simulink model "proiect_model2"  (R2023b)
settings: Solver=VariableStepAuto  StartTime=0.0  StopTime=30  RelTol=1e-3
settings Model: Creator=gabri  LastModifiedBy=gabri

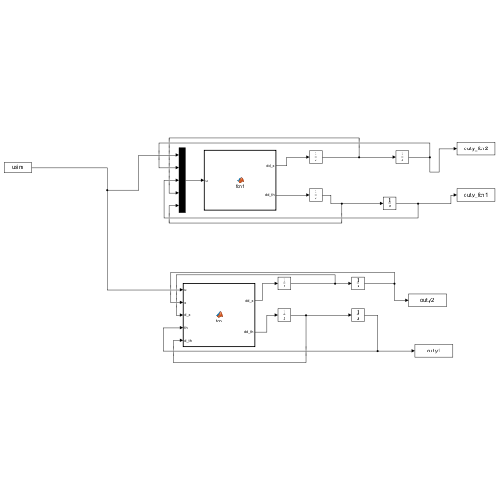
[thumbnail: Simulink's stored preview of the top-level diagram]
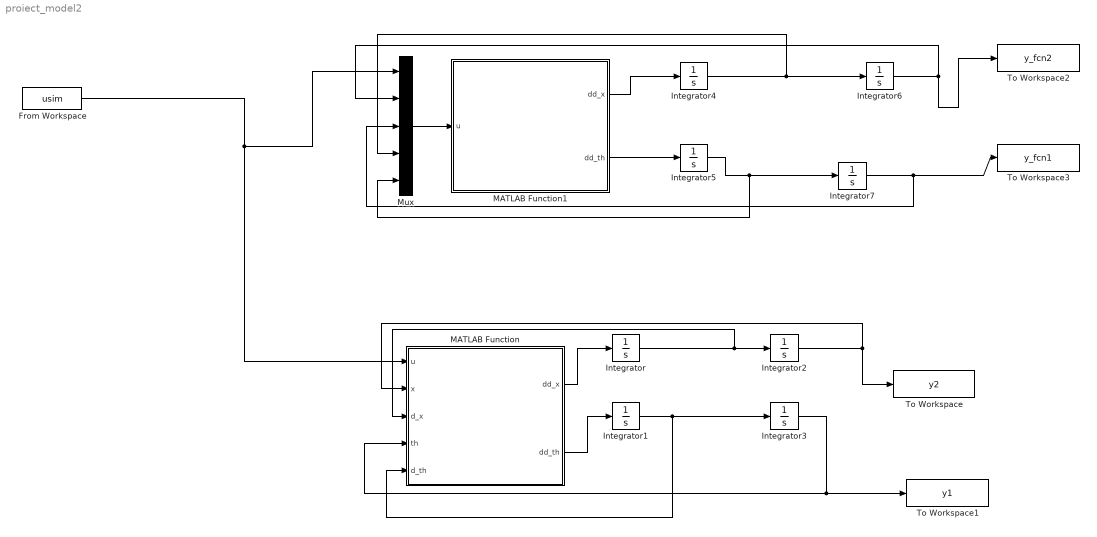
== system proiect_model2 ==
  From Workspace : FromWorkspace  VariableName=usim
  Integrator{,1..7} (8 alike) : Integrator
  MATLAB Function : MATLAB Function  TreatAsAtomicUnit=on
  MATLAB Function1 : MATLAB Function  TreatAsAtomicUnit=on
  Mux : Mux  Inputs=5
  To Workspace : ToWorkspace  VariableName=y2  SaveFormat=Timeseries  SampleTime=-1
      settings: Save2DSignal=2-D array (concatenate along first dimension)
  To Workspace1 : ToWorkspace  VariableName=y1  SaveFormat=Timeseries  SampleTime=-1
      settings: Save2DSignal=2-D array (concatenate along first dimension)
  To Workspace2 : ToWorkspace  VariableName=y_fcn2  SaveFormat=Timeseries  SampleTime=-1
      settings: Save2DSignal=2-D array (concatenate along first dimension)
  To Workspace3 : ToWorkspace  VariableName=y_fcn1  SaveFormat=Timeseries  SampleTime=-1
      settings: Save2DSignal=2-D array (concatenate along first dimension)
  wires:
  Integrator6/1 -> To Workspace2/1, Mux/2
  MATLAB Function/1(dd_x) -> Integrator/1
  Integrator7/1 -> To Workspace3/1, Mux/3
  MATLAB Function1/2(dd_th) -> Integrator5/1
  Mux/1 -> MATLAB Function1/1(u)
  Integrator4/1 -> Integrator6/1, Mux/4
  From Workspace/1 -> Mux/1, MATLAB Function/1(u)
  MATLAB Function1/1(dd_x) -> Integrator4/1
  Integrator5/1 -> Mux/5, Integrator7/1
  Integrator2/1 -> MATLAB Function/2(x), To Workspace/1
  Integrator1/1 -> Integrator3/1, MATLAB Function/5(d_th)
  Integrator3/1 -> To Workspace1/1, MATLAB Function/4(th)
  Integrator/1 -> MATLAB Function/3(d_x), Integrator2/1
  MATLAB Function/2(dd_th) -> Integrator1/1

== matlab function proiect_model2/MATLAB Function1 ==
  data: u input; dd_x output; dd_th output
function [dd_x, dd_th] = fcn1(u)

    %Alegerea valorilor pentru parametrii modelului in mod arbitrar(si pozitiv)
    l0 = 2.42;      %lungimea initiala
    m = 3.53;       %masa corpului   
    k = 3.21;       %constanta elastica
    fact = 0.61;    %factorul de amortizare
    g = 9.81;       %acceleratia gravitationala

    %Formulele modelului
    dd_x = (l0 + u(2)) * (u(5)) * (u(5)) - ((k *u(2)) / m) + g * cos(u(3)) - fact * u(4);
    dd_th = - (g * sin(u(3)) / (l0 + u(2)))- ((2 * u(4) * u(5)) / (l0 + u(2))) - fact * u(5) + (u(1) / (m * (l0 + u(2)) * (l0 + u(2))));

end

== matlab function proiect_model2/MATLAB Function ==
  data: dd_x output; u input; dd_th output; x input; d_x input; th input; d_th input
function [dd_x, dd_th] = fcn(u, x, d_x, th, d_th)
    
    %Alegerea valorilor pentru parametrii modelului in mod arbitrar(si pozitiv)
    l0 = 2.42;      %lungimea initiala
    m = 3.53;       %masa corpului   
    k = 3.21;       %constanta elastica
    fact = 0.61;    %factorul de amortizare
    g = 9.81;       %acceleratia gravitationala
    
    %Formulele modelului
    dd_x = (l0 + x) * (d_th) * (d_th) - ((k * x) / m) + g * cos(th) - fact * d_x;
    dd_th = - (g * sin(th)) / (l0 + x) - (2 * d_x / (l0 + x)) * d_th - fact * d_th + 1 / (m * (l0 + x) * (l0 + x)) * u;

end
